simulink model "planta_piloto"  (R2025b)
settings: Solver=VariableStepAuto  StartTime=0.0  StopTime=16  RelTol=1e-3
model workspace (MAT data in the model file):
  w = 0.5
undefined symbols (not defined in the file): C1, C2, C3, EV, GND, MTR, WHL
libraries: autolibutils x4, slpidlib x3, autolibmappedmotor x2, vehdynlibviscommon x1, vehdynlibdriver x1, autolibshared x1
(part 2 of 2)

== matlab function planta_piloto/MATLAB Function1 ==
  data: FL_speed input; FR_speed input; SR_L output; omega_RLwheel input; omega_RRwheel input; radius input; SR_R output
function [SR_L , SR_R] = fcn(FL_speed, FR_speed, omega_RLwheel, omega_RRwheel, radius)

SR_L = (omega_RLwheel * radius/FL_speed)-1;
SR_R = (omega_RRwheel * radius/FR_speed)-1;

== matlab function planta_piloto/MATLAB Function ==
  data: u input; y output
function y = fcn(u)

y = [u(1), u(2); u(3), u(4)];

== matlab function planta_piloto/MATLAB Function2 ==
  data: SR_L input; Atrito_L output; C1 input; C2 input; C3 input
function Atrito_L = fcn(SR_L, C1, C2, C3)

Atrito_L = (C1*(1-(exp(SR_L*C2*(-1)))))-(C3*SR_L);

== matlab function planta_piloto/MATLAB Function3 ==
  data: SR_R input; Atrito_R output; C1 input; C2 input; C3 input
function Atrito_R = fcn(SR_R, C1, C2, C3)

Atrito_R = (C1*(1-(exp(SR_R*C2*(-1)))))-(C3*SR_R);

== matlab function planta_piloto/MATLAB Function4 ==
  data: steering_angle input; desired_yaw output; Vcg input; Ku input; axles_dist input
function desired_yaw = fcn(steering_angle, Vcg, Ku, axles_dist)

desired_yaw = (Vcg*steering_angle)/(axles_dist+(Ku*Vcg*Vcg));

== matlab function planta_piloto/MATLAB Function5 ==
  data: angle input; atrito input; max_yaw output; Vcg input; g input; fi input
function max_yaw = fcn(angle, atrito, Vcg, g, fi)

if angle >= 0
    a = 1;
else
    a = -1;
end

max_yaw = a*(fi*atrito*g)/(Vcg);

== matlab function planta_piloto/MATLAB Function6 ==
  data: left_wheel_angle output; steering_angle input; right_wheel_angle output
function [left_wheel_angle, right_wheel_angle] = fcn(steering_angle)

if(steering_angle<=0)
    left_wheel_angle = 0.30732918494924799*steering_angle;
    right_wheel_angle = 0.268948751217872*steering_angle;

else (steering_angle>0)
    left_wheel_angle = 0.268948678266664*steering_angle;
    right_wheel_angle = 0.30732915888671*steering_angle;
end
end

== matlab function planta_piloto/MATLAB Function7 ==
  data: xdot input; Vx output; ydot input; Vy output; psi input
function [Vx, Vy] = fcn(xdot, ydot, psi)

Vx = (xdot*cos(psi)) + (ydot*sin(psi));
Vy = (xdot*sin(psi)) + (ydot*cos(psi));

== matlab function planta_piloto/MATLAB Function8 ==
  data: desired_yaw input; max_yaw input; VT_Setpoint output
function VT_Setpoint = fcn(desired_yaw, max_yaw)

if desired_yaw >= 0
    VT_Setpoint = min(desired_yaw, max_yaw);
else
    VT_Setpoint = max(desired_yaw, max_yaw);
end

== matlab function planta_piloto/MATLAB Function9 ==
  data: s input; x_ref output; R input; y_ref output; psi_ref output
function [x_ref, y_ref, psi_ref] = fcn(s, R)
%#codegen
% Esta função calcula as referências de trajetória para um círculo.
% - Início: [0, 0]
% - Centro: [R, 0]
% - Entrada s: Distância percorrida (do Integrator)
% - Entrada R: Raio do círculo (pode ser positivo ou negativo)
% - Saída x_ref: Posição X de referência
% - Saída y_ref: Posição Y de referência
% - Saída psi_ref: Ângulo da tangente (guinada de referência)

% 1. Definir o sinal do ângulo que fornecerá um erro inicial (seu sinal deve ser igual ao do raio)
if R >=0
    error = pi/5.5;
else
    error = -pi/5.5;
end

% 2. Calcular o ângulo do arco percorrido (theta)

if R == 0
    theta = 0; % Evita divisão por zero
else
    %esse pi/6 foi adicionado arbitrariamente. Sua função é fornecer um
    %erro inicial para o bloco do piloto, tornando a simulação mais
    %realista.
    theta = (s / R)+error;
end

% 3. Calcular a Posição de Referência (x_ref, y_ref) 
% OBS: X e Y são invertidos, é preciso tomar cuidado e o -1 é usado para
% ajustar a referência

y_ref = (R - R * cos(theta))*(-1);
x_ref = R * sin(theta);

% 4. Calcular o Ângulo de Referência (psi_ref)
% Este valor será atribuído diretamente à saída
% Usa a fórmula geométrica psi_ref = 90 - theta
psi_ref = - theta;

end
